simulink model "test_final_sift"  (R2015a)
settings: Solver=ode45  StartTime=0.0  StopTime=10.0  RelTol=1e-3
InitFcn:
  | %% DSPBuilder Start
  | alt_dspbuilder_update_model(bdroot)
  | %% DSPBuilder End
libraries: allblocks_alteradspbuilder2 x2309
(part 14 of 27)

== system test_final_sift/sift_octave1/matching/Ram/picture_first ==
  descriptor : Inport
  eof : Inport  Port=2
  clken : Inport  Port=3
  allow : Inport  Port=4
  AltBus : allblocks_alteradspbuilder2/AltBus  BusType=Unsigned Integer  bwl=1  bwr=0  saturate=off  floatingPointInput=on  floatingPointOutput=on  logOutputs=off  logFile=C:\Users\ASUS\Desktop\sift_fpga\Octave_2\tb_test_final_sift\test%5Ffinal%5Fsift_sift%5Foctave1_matching_Ram_picture%5Ffirst_AltBus.fixedpointlog
  AltBus1 : allblocks_alteradspbuilder2/AltBus  BusType=Unsigned Integer  bwl=1172  bwr=0  saturate=off  floatingPointInput=on  floatingPointOutput=on  logOutputs=off  logFile=C:\Users\ASUS\Desktop\sift_fpga\Octave_2\tb_test_final_sift\test%5Ffinal%5Fsift_sift%5Foctave1_matching_Ram_picture%5Ffirst_AltBus1.fixedpointlog
  Comparator : allblocks_alteradspbuilder2/Comparator  direction=a == b  pipeline_display=0  allowFloatingPointOverride=on  logOutputs=off  logFile=C:\Users\ASUS\Desktop\sift_fpga\Octave_2\tb_test_final_sift\test%5Ffinal%5Fsift_sift%5Foctave1_matching_Ram_picture%5Ffirst_Comparator.fixedpointlog
  Constant1 : allblocks_alteradspbuilder2/Constant  mask_cst=1  BusType=Single Bit  bwl=10  bwr=0  roundMode=Truncate  satMode=Wrap  SpecifyClock=off  allowFloatingPointOverride=on  logOutputs=off  logFile=C:\Users\ASUS\Desktop\sift_fpga\Octave_2\tb_test_final_sift\test%5Ffinal%5Fsift_sift%5Foctave1_matching_Ram_picture%5Ffirst_Constant1.fixedpointlog
  Constant2 : allblocks_alteradspbuilder2/Constant  mask_cst=1  BusType=Unsigned Integer  bwl=10  bwr=0  roundMode=Truncate  satMode=Wrap  SpecifyClock=off  allowFloatingPointOverride=on  logOutputs=off  logFile=C:\Users\ASUS\Desktop\sift_fpga\Octave_2\tb_test_final_sift\test%5Ffinal%5Fsift_sift%5Foctave1_matching_Ram_picture%5Ffirst_Constant2.fixedpointlog
  Constant3 : allblocks_alteradspbuilder2/Constant  mask_cst=1  BusType=Single Bit  bwl=1172  bwr=0  roundMode=Truncate  satMode=Wrap  SpecifyClock=off  allowFloatingPointOverride=on  logOutputs=off  logFile=C:\Users\ASUS\Desktop\sift_fpga\Octave_2\tb_test_final_sift\test%5Ffinal%5Fsift_sift%5Foctave1_matching_Ram_picture%5Ffirst_Constant3.fixedpointlog
  Constant4 : allblocks_alteradspbuilder2/Constant  mask_cst=1998  BusType=Unsigned Integer  bwl=1172  bwr=0  roundMode=Truncate  satMode=Wrap  SpecifyClock=off  allowFloatingPointOverride=on  logOutputs=off  logFile=C:\Users\ASUS\Desktop\sift_fpga\Octave_2\tb_test_final_sift\test%5Ffinal%5Fsift_sift%5Foctave1_matching_Ram_picture%5Ffirst_Constant4.fixedpointlog
  Counter : allblocks_alteradspbuilder2/Counter  BusType=Unsigned Integer  bwl=10  bwr=0  use_modulo=on  modulo=1000  SpecifyClock=off  direction=Increment  use_sload=off  use_sset=off  svalue=1  use_clk_ena=off  use_ena=on  use_sclr=on  pipeline_display=1
  Delay : allblocks_alteradspbuilder2/Delay  pipeline=1  pipeline_display=1  ClockPhase=1  use_ena=on  use_sclr=off  allowFloatingPointOverride=on  logOutputs=off  logFile=C:\Users\ASUS\Desktop\sift_fpga\Octave_2\tb_test_final_sift\test%5Ffinal%5Fsift_sift%5Foctave1_matching_Ram_picture%5Ffirst_Delay.fixedpointlog  use_init=off  reset_value=1
  Delay1 : allblocks_alteradspbuilder2/Delay  pipeline=1  pipeline_display=1  ClockPhase=1  use_ena=on  use_sclr=off  allowFloatingPointOverride=on  logOutputs=off  logFile=C:\Users\ASUS\Desktop\sift_fpga\Octave_2\tb_test_final_sift\test%5Ffinal%5Fsift_sift%5Foctave1_matching_Ram_picture%5Ffirst_Delay1.fixedpointlog  use_init=off  reset_value=1
  Delay2 : allblocks_alteradspbuilder2/Delay  pipeline=1  pipeline_display=1  ClockPhase=1  use_ena=on  use_sclr=off  allowFloatingPointOverride=on  logOutputs=off  logFile=C:\Users\ASUS\Desktop\sift_fpga\Octave_2\tb_test_final_sift\test%5Ffinal%5Fsift_sift%5Foctave1_matching_Ram_picture%5Ffirst_Delay2.fixedpointlog  use_init=off  reset_value=1
  Delay3 : allblocks_alteradspbuilder2/Delay  pipeline=1  pipeline_display=1  ClockPhase=1  use_ena=on  use_sclr=off  allowFloatingPointOverride=on  logOutputs=off  logFile=C:\Users\ASUS\Desktop\sift_fpga\Octave_2\tb_test_final_sift\test%5Ffinal%5Fsift_sift%5Foctave1_matching_Ram_picture%5Ffirst_Delay3.fixedpointlog  use_init=off  reset_value=1
  Delay4 : allblocks_alteradspbuilder2/Delay  pipeline=1  pipeline_display=1  ClockPhase=1  use_ena=on  use_sclr=off  allowFloatingPointOverride=on  logOutputs=off  logFile=C:\Users\ASUS\Desktop\sift_fpga\Octave_2\tb_test_final_sift\test%5Ffinal%5Fsift_sift%5Foctave1_matching_Ram_picture%5Ffirst_Delay4.fixedpointlog  use_init=off  reset_value=1
  Logical Bit Operator : allblocks_alteradspbuilder2/Logical Bit Operator  LogicalOperator=OR  user_inputs=2  pipeline_display=0
  Logical Bit Operator1 : allblocks_alteradspbuilder2/Logical Bit Operator  LogicalOperator=AND  user_inputs=2  pipeline_display=0
  Logical Bit Operator2 : allblocks_alteradspbuilder2/Logical Bit Operator  LogicalOperator=NAND  user_inputs=2  pipeline_display=0
  Logical Bit Operator3 : allblocks_alteradspbuilder2/Logical Bit Operator  LogicalOperator=AND  user_inputs=2  pipeline_display=0
  Logical Bus Operator : allblocks_alteradspbuilder2/Logical Bus Operator  BusType=Unsigned Integer  bwl=1173  bwr=0  LogicalOp_text=Shift Right  mask_value_num=-5  shift_amount=1172  force_sign_ext=off  pipeline_display=0
  Multiplexer : allblocks_alteradspbuilder2/Multiplexer  numInputs=2  pipeline=0  oneHot=off  pipeline_display=0  use_ena=off  use_aclr=off  allowFloatingPointOverride=on  logOutputs=off  logFile=C:\Users\ASUS\Desktop\sift_fpga\Octave_2\tb_test_final_sift\test%5Ffinal%5Fsift_sift%5Foctave1_matching_Ram_picture%5Ffirst_Multiplexer.fixedpointlog
  Multiplexer1 : allblocks_alteradspbuilder2/Multiplexer  numInputs=2  pipeline=0  oneHot=off  pipeline_display=0  use_ena=off  use_aclr=off  allowFloatingPointOverride=on  logOutputs=off  logFile=C:\Users\ASUS\Desktop\sift_fpga\Octave_2\tb_test_final_sift\test%5Ffinal%5Fsift_sift%5Foctave1_matching_Ram_picture%5Ffirst_Multiplexer1.fixedpointlog
  Multiplexer2 : allblocks_alteradspbuilder2/Multiplexer  numInputs=2  pipeline=0  oneHot=off  pipeline_display=0  use_ena=off  use_aclr=off  allowFloatingPointOverride=on  logOutputs=off  logFile=C:\Users\ASUS\Desktop\sift_fpga\Octave_2\tb_test_final_sift\test%5Ffinal%5Fsift_sift%5Foctave1_matching_Ram_picture%5Ffirst_Multiplexer2.fixedpointlog
  Parallel Adder Subtractor : allblocks_alteradspbuilder2/Parallel Adder Subtractor  number_of_inputs=2  direction=+  use_pipeline=on  pipeline_display=1  phase_selection=1  use_ena=on  use_aclr=off  allowFloatingPointOverride=on  logOutputs=off  logFile=C:\Users\ASUS\Desktop\sift_fpga\Octave_2\tb_test_final_sift\test%5Ffinal%5Fsift_sift%5Foctave1_matching_Ram_picture%5Ffirst_Parallel+Adder+Subtractor.fixedpointlog
  data : Outport
  add_write : Outport  Port=2
  ena_write : Outport  Port=3
  wires:
  descriptor/1 -> [descriptor]
  [descriptor] -> Logical Bus Operator/1
  Logical Bus Operator/1 -> AltBus/1
  AltBus/1 -> [isKeyPoint]
  [isKeyPoint] -> Logical Bit Operator/1
  eof/1 -> [eof]
  [eof] -> Delay4/1
  Counter/1 -> [add_write]
  [descriptor] -> AltBus1/1
  AltBus1/1 -> [data]
  [eof] -> Comparator/1
  Constant1/1 -> Comparator/2
  [sel] -> Multiplexer/1
  Multiplexer/1 -> Delay1/1
  Comparator/1 -> [sel]
  [data] -> Multiplexer/2
  Constant4/1 -> Multiplexer/3
  clken/1 -> [clken]
  Delay1/1 -> data/1
  [ena] -> Delay1/2
  [sel] -> Delay3/1
  [add_write] -> Delay/1
  Multiplexer1/1 -> add_write/1
  Delay/1 -> Multiplexer1/2
  [ena] -> Delay/2
  [add_write] -> Parallel Adder Subtractor/1
  Constant2/1 -> Parallel Adder Subtractor/2
  [ena] -> Parallel Adder Subtractor/3
  Parallel Adder Subtractor/1 -> Multiplexer1/3
  [sel] -> Multiplexer2/1
  Multiplexer2/1 -> Delay2/1
  [isKeyPoint] -> Multiplexer2/2
  Constant3/1 -> Multiplexer2/3
  [ena] -> Delay2/2
  Delay3/1 -> Multiplexer1/1
  [ena] -> Delay3/2
  Logical Bit Operator/1 -> Counter/1
  Delay4/1 -> Counter/2, Logical Bit Operator/2
  [ena] -> Delay4/2
  allow/1 -> [allow]
  [allow] -> Logical Bit Operator2/2, Logical Bit Operator2/1
  [clken] -> Logical Bit Operator1/2
  Logical Bit Operator2/1 -> Logical Bit Operator1/1
  Logical Bit Operator1/1 -> [ena]
  Delay2/1 -> Logical Bit Operator3/1
  Logical Bit Operator3/1 -> ena_write/1
  [ena] -> Logical Bit Operator3/2

== system test_final_sift/sift_octave1/matching/Ram/picture_second ==
  descriptor : Inport
  eof : Inport  Port=2
  clken : Inport  Port=3
  allow : Inport  Port=4
  AltBus : allblocks_alteradspbuilder2/AltBus  BusType=Unsigned Integer  bwl=1  bwr=0  saturate=off  floatingPointInput=on  floatingPointOutput=on  logOutputs=off  logFile=C:\Users\ASUS\Desktop\sift_fpga\Octave_2\tb_test_final_sift\test%5Ffinal%5Fsift_sift%5Foctave1_matching_Ram_picture%5Fsecond_AltBus.fixedpointlog
  AltBus1 : allblocks_alteradspbuilder2/AltBus  BusType=Unsigned Integer  bwl=1172  bwr=0  saturate=off  floatingPointInput=on  floatingPointOutput=on  logOutputs=off  logFile=C:\Users\ASUS\Desktop\sift_fpga\Octave_2\tb_test_final_sift\test%5Ffinal%5Fsift_sift%5Foctave1_matching_Ram_picture%5Fsecond_AltBus1.fixedpointlog
  Comparator : allblocks_alteradspbuilder2/Comparator  direction=a == b  pipeline_display=0  allowFloatingPointOverride=on  logOutputs=off  logFile=C:\Users\ASUS\Desktop\sift_fpga\Octave_2\tb_test_final_sift\test%5Ffinal%5Fsift_sift%5Foctave1_matching_Ram_picture%5Fsecond_Comparator.fixedpointlog
  Constant1 : allblocks_alteradspbuilder2/Constant  mask_cst=1  BusType=Single Bit  bwl=10  bwr=0  roundMode=Truncate  satMode=Wrap  SpecifyClock=off  allowFloatingPointOverride=on  logOutputs=off  logFile=C:\Users\ASUS\Desktop\sift_fpga\Octave_2\tb_test_final_sift\test%5Ffinal%5Fsift_sift%5Foctave1_matching_Ram_picture%5Fsecond_Constant1.fixedpointlog
  Constant2 : allblocks_alteradspbuilder2/Constant  mask_cst=1  BusType=Unsigned Integer  bwl=10  bwr=0  roundMode=Truncate  satMode=Wrap  SpecifyClock=off  allowFloatingPointOverride=on  logOutputs=off  logFile=C:\Users\ASUS\Desktop\sift_fpga\Octave_2\tb_test_final_sift\test%5Ffinal%5Fsift_sift%5Foctave1_matching_Ram_picture%5Fsecond_Constant2.fixedpointlog
  Constant3 : allblocks_alteradspbuilder2/Constant  mask_cst=1  BusType=Single Bit  bwl=1172  bwr=0  roundMode=Truncate  satMode=Wrap  SpecifyClock=off  allowFloatingPointOverride=on  logOutputs=off  logFile=C:\Users\ASUS\Desktop\sift_fpga\Octave_2\tb_test_final_sift\test%5Ffinal%5Fsift_sift%5Foctave1_matching_Ram_picture%5Fsecond_Constant3.fixedpointlog
  Constant4 : allblocks_alteradspbuilder2/Constant  mask_cst=1998  BusType=Unsigned Integer  bwl=1172  bwr=0  roundMode=Truncate  satMode=Wrap  SpecifyClock=off  allowFloatingPointOverride=on  logOutputs=off  logFile=C:\Users\ASUS\Desktop\sift_fpga\Octave_2\tb_test_final_sift\test%5Ffinal%5Fsift_sift%5Foctave1_matching_Ram_picture%5Fsecond_Constant4.fixedpointlog
  Counter : allblocks_alteradspbuilder2/Counter  BusType=Unsigned Integer  bwl=10  bwr=0  use_modulo=on  modulo=1000  SpecifyClock=off  direction=Increment  use_sload=off  use_sset=off  svalue=1  use_clk_ena=off  use_ena=on  use_sclr=on  pipeline_display=1
  Delay : allblocks_alteradspbuilder2/Delay  pipeline=1  pipeline_display=1  ClockPhase=1  use_ena=on  use_sclr=off  allowFloatingPointOverride=on  logOutputs=off  logFile=C:\Users\ASUS\Desktop\sift_fpga\Octave_2\tb_test_final_sift\test%5Ffinal%5Fsift_sift%5Foctave1_matching_Ram_picture%5Fsecond_Delay.fixedpointlog  use_init=off  reset_value=1
  Delay1 : allblocks_alteradspbuilder2/Delay  pipeline=1  pipeline_display=1  ClockPhase=1  use_ena=on  use_sclr=off  allowFloatingPointOverride=on  logOutputs=off  logFile=C:\Users\ASUS\Desktop\sift_fpga\Octave_2\tb_test_final_sift\test%5Ffinal%5Fsift_sift%5Foctave1_matching_Ram_picture%5Fsecond_Delay1.fixedpointlog  use_init=off  reset_value=1
  Delay2 : allblocks_alteradspbuilder2/Delay  pipeline=1  pipeline_display=1  ClockPhase=1  use_ena=on  use_sclr=off  allowFloatingPointOverride=on  logOutputs=off  logFile=C:\Users\ASUS\Desktop\sift_fpga\Octave_2\tb_test_final_sift\test%5Ffinal%5Fsift_sift%5Foctave1_matching_Ram_picture%5Fsecond_Delay2.fixedpointlog  use_init=off  reset_value=1
  Delay3 : allblocks_alteradspbuilder2/Delay  pipeline=1  pipeline_display=1  ClockPhase=1  use_ena=on  use_sclr=off  allowFloatingPointOverride=on  logOutputs=off  logFile=C:\Users\ASUS\Desktop\sift_fpga\Octave_2\tb_test_final_sift\test%5Ffinal%5Fsift_sift%5Foctave1_matching_Ram_picture%5Fsecond_Delay3.fixedpointlog  use_init=off  reset_value=1
  Delay4 : allblocks_alteradspbuilder2/Delay  pipeline=1  pipeline_display=1  ClockPhase=1  use_ena=on  use_sclr=off  allowFloatingPointOverride=on  logOutputs=off  logFile=C:\Users\ASUS\Desktop\sift_fpga\Octave_2\tb_test_final_sift\test%5Ffinal%5Fsift_sift%5Foctave1_matching_Ram_picture%5Fsecond_Delay4.fixedpointlog  use_init=off  reset_value=1
  Logical Bit Operator : allblocks_alteradspbuilder2/Logical Bit Operator  LogicalOperator=OR  user_inputs=2  pipeline_display=0
  Logical Bit Operator1 : allblocks_alteradspbuilder2/Logical Bit Operator  LogicalOperator=AND  user_inputs=2  pipeline_display=0
  Logical Bit Operator3 : allblocks_alteradspbuilder2/Logical Bit Operator  LogicalOperator=AND  user_inputs=2  pipeline_display=0
  Logical Bus Operator : allblocks_alteradspbuilder2/Logical Bus Operator  BusType=Unsigned Integer  bwl=1173  bwr=0  LogicalOp_text=Shift Right  mask_value_num=-5  shift_amount=1172  force_sign_ext=off  pipeline_display=0
  Multiplexer : allblocks_alteradspbuilder2/Multiplexer  numInputs=2  pipeline=0  oneHot=off  pipeline_display=0  use_ena=off  use_aclr=off  allowFloatingPointOverride=on  logOutputs=off  logFile=C:\Users\ASUS\Desktop\sift_fpga\Octave_2\tb_test_final_sift\test%5Ffinal%5Fsift_sift%5Foctave1_matching_Ram_picture%5Fsecond_Multiplexer.fixedpointlog
  Multiplexer1 : allblocks_alteradspbuilder2/Multiplexer  numInputs=2  pipeline=0  oneHot=off  pipeline_display=0  use_ena=off  use_aclr=off  allowFloatingPointOverride=on  logOutputs=off  logFile=C:\Users\ASUS\Desktop\sift_fpga\Octave_2\tb_test_final_sift\test%5Ffinal%5Fsift_sift%5Foctave1_matching_Ram_picture%5Fsecond_Multiplexer1.fixedpointlog
  Multiplexer2 : allblocks_alteradspbuilder2/Multiplexer  numInputs=2  pipeline=0  oneHot=off  pipeline_display=0  use_ena=off  use_aclr=off  allowFloatingPointOverride=on  logOutputs=off  logFile=C:\Users\ASUS\Desktop\sift_fpga\Octave_2\tb_test_final_sift\test%5Ffinal%5Fsift_sift%5Foctave1_matching_Ram_picture%5Fsecond_Multiplexer2.fixedpointlog
  Parallel Adder Subtractor : allblocks_alteradspbuilder2/Parallel Adder Subtractor  number_of_inputs=2  direction=+  use_pipeline=on  pipeline_display=1  phase_selection=1  use_ena=on  use_aclr=off  allowFloatingPointOverride=on  logOutputs=off  logFile=C:\Users\ASUS\Desktop\sift_fpga\Octave_2\tb_test_final_sift\test%5Ffinal%5Fsift_sift%5Foctave1_matching_Ram_picture%5Fsecond_Parallel+Adder+Subtractor.fixedpointlog
  data : Outport
  add_write : Outport  Port=2
  ena_write : Outport  Port=3
  wires:
  descriptor/1 -> [descriptor]
  [descriptor] -> Logical Bus Operator/1
  Logical Bus Operator/1 -> AltBus/1
  AltBus/1 -> [isKeyPoint]
  [isKeyPoint] -> Logical Bit Operator/1
  eof/1 -> [eof]
  [eof] -> Delay4/1
  Counter/1 -> [add_write]
  [descriptor] -> AltBus1/1
  AltBus1/1 -> [data]
  [eof] -> Comparator/1
  Constant1/1 -> Comparator/2
  [sel] -> Multiplexer/1
  Multiplexer/1 -> Delay1/1
  Comparator/1 -> [sel]
  [data] -> Multiplexer/2
  Constant4/1 -> Multiplexer/3
  clken/1 -> [clken]
  Delay1/1 -> data/1
  [ena] -> Delay1/2
  [sel] -> Delay3/1
  [add_write] -> Delay/1
  Multiplexer1/1 -> add_write/1
  Delay/1 -> Multiplexer1/2
  [ena] -> Delay/2
  [add_write] -> Parallel Adder Subtractor/1
  Constant2/1 -> Parallel Adder Subtractor/2
  [ena] -> Parallel Adder Subtractor/3
  Parallel Adder Subtractor/1 -> Multiplexer1/3
  [sel] -> Multiplexer2/1
  Multiplexer2/1 -> Delay2/1
  [isKeyPoint] -> Multiplexer2/2
  Constant3/1 -> Multiplexer2/3
  [ena] -> Delay2/2
  Delay3/1 -> Multiplexer1/1
  [ena] -> Delay3/2
  Logical Bit Operator/1 -> Counter/1
  Delay4/1 -> Counter/2, Logical Bit Operator/2
  [ena] -> Delay4/2
  allow/1 -> [allow]
  [allow] -> Logical Bit Operator1/1
  [clken] -> Logical Bit Operator1/2
  Logical Bit Operator1/1 -> [ena]
  Delay2/1 -> Logical Bit Operator3/1
  Logical Bit Operator3/1 -> ena_write/1
  [ena] -> Logical Bit Operator3/2

== system test_final_sift/sift_octave1/matching/compare_descriptor/BusSplitter ==
  descriptor_in : Inport
  AltBus : allblocks_alteradspbuilder2/AltBus  BusType=Unsigned Integer  bwl=1024  bwr=0  saturate=off  floatingPointInput=on  floatingPointOutput=on  logOutputs=off  logFile=C:\Users\ASUS\Desktop\sift_fpga\Octave_2\tb_test_final_sift\test%5Ffinal%5Fsift_sift%5Foctave1_matching_compare%5Fdescriptor_BusSplitter_AltBus.fixedpointlog
  AltBus1 : allblocks_alteradspbuilder2/AltBus  BusType=Unsigned Integer  bwl=896  bwr=0  saturate=off  floatingPointInput=on  floatingPointOutput=on  logOutputs=off  logFile=C:\Users\ASUS\Desktop\sift_fpga\Octave_2\tb_test_final_sift\test%5Ffinal%5Fsift_sift%5Foctave1_matching_compare%5Fdescriptor_BusSplitter_AltBus1.fixedpointlog
  AltBus10 : allblocks_alteradspbuilder2/AltBus  BusType=Unsigned Integer  bwl=128  bwr=0  saturate=off  floatingPointInput=on  floatingPointOutput=on  logOutputs=off  logFile=C:\Users\ASUS\Desktop\sift_fpga\Octave_2\tb_test_final_sift\test%5Ffinal%5Fsift_sift%5Foctave1_matching_compare%5Fdescriptor_BusSplitter_AltBus10.fixedpointlog
  AltBus11 : allblocks_alteradspbuilder2/AltBus  BusType=Unsigned Integer  bwl=128  bwr=0  saturate=off  floatingPointInput=on  floatingPointOutput=on  logOutputs=off  logFile=C:\Users\ASUS\Desktop\sift_fpga\Octave_2\tb_test_final_sift\test%5Ffinal%5Fsift_sift%5Foctave1_matching_compare%5Fdescriptor_BusSplitter_AltBus11.fixedpointlog
  AltBus12 : allblocks_alteradspbuilder2/AltBus  BusType=Unsigned Integer  bwl=128  bwr=0  saturate=off  floatingPointInput=on  floatingPointOutput=on  logOutputs=off  logFile=C:\Users\ASUS\Desktop\sift_fpga\Octave_2\tb_test_final_sift\test%5Ffinal%5Fsift_sift%5Foctave1_matching_compare%5Fdescriptor_BusSplitter_AltBus12.fixedpointlog
  AltBus13 : allblocks_alteradspbuilder2/AltBus  BusType=Unsigned Integer  bwl=128  bwr=0  saturate=off  floatingPointInput=on  floatingPointOutput=on  logOutputs=off  logFile=C:\Users\ASUS\Desktop\sift_fpga\Octave_2\tb_test_final_sift\test%5Ffinal%5Fsift_sift%5Foctave1_matching_compare%5Fdescriptor_BusSplitter_AltBus13.fixedpointlog
  AltBus14 : allblocks_alteradspbuilder2/AltBus  BusType=Unsigned Integer  bwl=16*8*9  bwr=0  saturate=off  floatingPointInput=on  floatingPointOutput=on  logOutputs=off  logFile=C:\Users\ASUS\Desktop\sift_fpga\Octave_2\tb_test_final_sift\test%5Ffinal%5Fsift_sift%5Foctave1_matching_compare%5Fdescriptor_BusSplitter_AltBus14.fixedpointlog
  AltBus15 : allblocks_alteradspbuilder2/AltBus  BusType=Unsigned Integer  bwl=128  bwr=0  saturate=off  floatingPointInput=on  floatingPointOutput=on  logOutputs=off  logFile=C:\Users\ASUS\Desktop\sift_fpga\Octave_2\tb_test_final_sift\test%5Ffinal%5Fsift_sift%5Foctave1_matching_compare%5Fdescriptor_BusSplitter_AltBus15.fixedpointlog
  AltBus16 : allblocks_alteradspbuilder2/AltBus  BusType=Unsigned Integer  bwl=256  bwr=0  saturate=off  floatingPointInput=on  floatingPointOutput=on  logOutputs=off  logFile=C:\Users\ASUS\Desktop\sift_fpga\Octave_2\tb_test_final_sift\test%5Ffinal%5Fsift_sift%5Foctave1_matching_compare%5Fdescriptor_BusSplitter_AltBus16.fixedpointlog
  AltBus2 : allblocks_alteradspbuilder2/AltBus  BusType=Unsigned Integer  bwl=768  bwr=0  saturate=off  floatingPointInput=on  floatingPointOutput=on  logOutputs=off  logFile=C:\Users\ASUS\Desktop\sift_fpga\Octave_2\tb_test_final_sift\test%5Ffinal%5Fsift_sift%5Foctave1_matching_compare%5Fdescriptor_BusSplitter_AltBus2.fixedpointlog
  AltBus3 : allblocks_alteradspbuilder2/AltBus  BusType=Unsigned Integer  bwl=640  bwr=0  saturate=off  floatingPointInput=on  floatingPointOutput=on  logOutputs=off  logFile=C:\Users\ASUS\Desktop\sift_fpga\Octave_2\tb_test_final_sift\test%5Ffinal%5Fsift_sift%5Foctave1_matching_compare%5Fdescriptor_BusSplitter_AltBus3.fixedpointlog
  AltBus4 : allblocks_alteradspbuilder2/AltBus  BusType=Unsigned Integer  bwl=512  bwr=0  saturate=off  floatingPointInput=on  floatingPointOutput=on  logOutputs=off  logFile=C:\Users\ASUS\Desktop\sift_fpga\Octave_2\tb_test_final_sift\test%5Ffinal%5Fsift_sift%5Foctave1_matching_compare%5Fdescriptor_BusSplitter_AltBus4.fixedpointlog
  AltBus5 : allblocks_alteradspbuilder2/AltBus  BusType=Unsigned Integer  bwl=384  bwr=0  saturate=off  floatingPointInput=on  floatingPointOutput=on  logOutputs=off  logFile=C:\Users\ASUS\Desktop\sift_fpga\Octave_2\tb_test_final_sift\test%5Ffinal%5Fsift_sift%5Foctave1_matching_compare%5Fdescriptor_BusSplitter_AltBus5.fixedpointlog
  AltBus6 : allblocks_alteradspbuilder2/AltBus  BusType=Unsigned Integer  bwl=128  bwr=0  saturate=off  floatingPointInput=on  floatingPointOutput=on  logOutputs=off  logFile=C:\Users\ASUS\Desktop\sift_fpga\Octave_2\tb_test_final_sift\test%5Ffinal%5Fsift_sift%5Foctave1_matching_compare%5Fdescriptor_BusSplitter_AltBus6.fixedpointlog
  AltBus7 : allblocks_alteradspbuilder2/AltBus  BusType=Unsigned Integer  bwl=128  bwr=0  saturate=off  floatingPointInput=on  floatingPointOutput=on  logOutputs=off  logFile=C:\Users\ASUS\Desktop\sift_fpga\Octave_2\tb_test_final_sift\test%5Ffinal%5Fsift_sift%5Foctave1_matching_compare%5Fdescriptor_BusSplitter_AltBus7.fixedpointlog
  AltBus8 : allblocks_alteradspbuilder2/AltBus  BusType=Unsigned Integer  bwl=128  bwr=0  saturate=off  floatingPointInput=on  floatingPointOutput=on  logOutputs=off  logFile=C:\Users\ASUS\Desktop\sift_fpga\Octave_2\tb_test_final_sift\test%5Ffinal%5Fsift_sift%5Foctave1_matching_compare%5Fdescriptor_BusSplitter_AltBus8.fixedpointlog
  AltBus9 : allblocks_alteradspbuilder2/AltBus  BusType=Unsigned Integer  bwl=128  bwr=0  saturate=off  floatingPointInput=on  floatingPointOutput=on  logOutputs=off  logFile=C:\Users\ASUS\Desktop\sift_fpga\Octave_2\tb_test_final_sift\test%5Ffinal%5Fsift_sift%5Foctave1_matching_compare%5Fdescriptor_BusSplitter_AltBus9.fixedpointlog
  Logical Bus Operator : allblocks_alteradspbuilder2/Logical Bus Operator  BusType=Unsigned Integer  bwl=1152  bwr=0  LogicalOp_text=Shift Right  mask_value_num=-5  shift_amount=8*128  force_sign_ext=off  pipeline_display=0
  Logical Bus Operator1 : allblocks_alteradspbuilder2/Logical Bus Operator  BusType=Unsigned Integer  bwl=1024  bwr=0  LogicalOp_text=Shift Right  mask_value_num=-5  shift_amount=7*128  force_sign_ext=off  pipeline_display=0
  Logical Bus Operator2 : allblocks_alteradspbuilder2/Logical Bus Operator  BusType=Unsigned Integer  bwl=896  bwr=0  LogicalOp_text=Shift Right  mask_value_num=-5  shift_amount=6*128  force_sign_ext=off  pipeline_display=0
  Logical Bus Operator3 : allblocks_alteradspbuilder2/Logical Bus Operator  BusType=Unsigned Integer  bwl=768  bwr=0  LogicalOp_text=Shift Right  mask_value_num=-5  shift_amount=5*128  force_sign_ext=off  pipeline_display=0
  Logical Bus Operator4 : allblocks_alteradspbuilder2/Logical Bus Operator  BusType=Unsigned Integer  bwl=640  bwr=0  LogicalOp_text=Shift Right  mask_value_num=-5  shift_amount=4*128  force_sign_ext=off  pipeline_display=0
  Logical Bus Operator5 : allblocks_alteradspbuilder2/Logical Bus Operator  BusType=Unsigned Integer  bwl=512  bwr=0  LogicalOp_text=Shift Right  mask_value_num=-5  shift_amount=3*128  force_sign_ext=off  pipeline_display=0
  Logical Bus Operator6 : allblocks_alteradspbuilder2/Logical Bus Operator  BusType=Unsigned Integer  bwl=384  bwr=0  LogicalOp_text=Shift Right  mask_value_num=-5  shift_amount=2*128  force_sign_ext=off  pipeline_display=0
  Logical Bus Operator7 : allblocks_alteradspbuilder2/Logical Bus Operator  BusType=Unsigned Integer  bwl=256  bwr=0  LogicalOp_text=Shift Right  mask_value_num=-5  shift_amount=128  force_sign_ext=off  pipeline_display=0
  hist1 : Outport
  hist2 : Outport  Port=2
  hist3 : Outport  Port=3
  hist4 : Outport  Port=4
  hist5 : Outport  Port=5
  hist6 : Outport  Port=6
  hist7 : Outport  Port=7
  hist8 : Outport  Port=8
  hist9 : Outport  Port=9
  wires:
  Logical Bus Operator6/1 -> AltBus7/1
  AltBus1/1 -> Logical Bus Operator2/1
  AltBus9/1 -> hist5/1
  AltBus8/1 -> hist6/1
  AltBus7/1 -> hist7/1
  AltBus6/1 -> hist8/1
  AltBus/1 -> Logical Bus Operator1/1
  AltBus10/1 -> hist4/1
  AltBus12/1 -> hist3/1
  AltBus11/1 -> hist1/1
  AltBus3/1 -> Logical Bus Operator4/1
  AltBus2/1 -> Logical Bus Operator3/1
  AltBus4/1 -> Logical Bus Operator5/1
  descriptor_in/1 -> AltBus14/1
  AltBus5/1 -> Logical Bus Operator6/1
  Logical Bus Operator1/1 -> AltBus13/1
  Logical Bus Operator2/1 -> AltBus12/1
  Logical Bus Operator/1 -> AltBus11/1
  Logical Bus Operator5/1 -> AltBus8/1
  Logical Bus Operator4/1 -> AltBus9/1
  Logical Bus Operator3/1 -> AltBus10/1
  AltBus13/1 -> hist2/1
  AltBus15/1 -> hist9/1
  AltBus14/1 -> AltBus15/1, AltBus16/1, AltBus5/1, AltBus4/1, AltBus3/1, AltBus2/1, AltBus1/1, AltBus/1, Logical Bus Operator/1
  AltBus16/1 -> Logical Bus Operator7/1
  Logical Bus Operator7/1 -> AltBus6/1

== system test_final_sift/sift_octave1/matching/compare_descriptor/BusSplitter1 ==
  descriptor_in : Inport
  AltBus : allblocks_alteradspbuilder2/AltBus  BusType=Unsigned Integer  bwl=1024  bwr=0  saturate=off  floatingPointInput=on  floatingPointOutput=on  logOutputs=off  logFile=C:\Users\ASUS\Desktop\sift_fpga\Octave_2\tb_test_final_sift\test%5Ffinal%5Fsift_sift%5Foctave1_matching_compare%5Fdescriptor_BusSplitter1_AltBus.fixedpointlog
  AltBus1 : allblocks_alteradspbuilder2/AltBus  BusType=Unsigned Integer  bwl=896  bwr=0  saturate=off  floatingPointInput=on  floatingPointOutput=on  logOutputs=off  logFile=C:\Users\ASUS\Desktop\sift_fpga\Octave_2\tb_test_final_sift\test%5Ffinal%5Fsift_sift%5Foctave1_matching_compare%5Fdescriptor_BusSplitter1_AltBus1.fixedpointlog
  AltBus10 : allblocks_alteradspbuilder2/AltBus  BusType=Unsigned Integer  bwl=128  bwr=0  saturate=off  floatingPointInput=on  floatingPointOutput=on  logOutputs=off  logFile=C:\Users\ASUS\Desktop\sift_fpga\Octave_2\tb_test_final_sift\test%5Ffinal%5Fsift_sift%5Foctave1_matching_compare%5Fdescriptor_BusSplitter1_AltBus10.fixedpointlog
  AltBus11 : allblocks_alteradspbuilder2/AltBus  BusType=Unsigned Integer  bwl=128  bwr=0  saturate=off  floatingPointInput=on  floatingPointOutput=on  logOutputs=off  logFile=C:\Users\ASUS\Desktop\sift_fpga\Octave_2\tb_test_final_sift\test%5Ffinal%5Fsift_sift%5Foctave1_matching_compare%5Fdescriptor_BusSplitter1_AltBus11.fixedpointlog
  AltBus12 : allblocks_alteradspbuilder2/AltBus  BusType=Unsigned Integer  bwl=128  bwr=0  saturate=off  floatingPointInput=on  floatingPointOutput=on  logOutputs=off  logFile=C:\Users\ASUS\Desktop\sift_fpga\Octave_2\tb_test_final_sift\test%5Ffinal%5Fsift_sift%5Foctave1_matching_compare%5Fdescriptor_BusSplitter1_AltBus12.fixedpointlog
  AltBus13 : allblocks_alteradspbuilder2/AltBus  BusType=Unsigned Integer  bwl=128  bwr=0  saturate=off  floatingPointInput=on  floatingPointOutput=on  logOutputs=off  logFile=C:\Users\ASUS\Desktop\sift_fpga\Octave_2\tb_test_final_sift\test%5Ffinal%5Fsift_sift%5Foctave1_matching_compare%5Fdescriptor_BusSplitter1_AltBus13.fixedpointlog
  AltBus14 : allblocks_alteradspbuilder2/AltBus  BusType=Unsigned Integer  bwl=16*8*9  bwr=0  saturate=off  floatingPointInput=on  floatingPointOutput=on  logOutputs=off  logFile=C:\Users\ASUS\Desktop\sift_fpga\Octave_2\tb_test_final_sift\test%5Ffinal%5Fsift_sift%5Foctave1_matching_compare%5Fdescriptor_BusSplitter1_AltBus14.fixedpointlog
  AltBus15 : allblocks_alteradspbuilder2/AltBus  BusType=Unsigned Integer  bwl=128  bwr=0  saturate=off  floatingPointInput=on  floatingPointOutput=on  logOutputs=off  logFile=C:\Users\ASUS\Desktop\sift_fpga\Octave_2\tb_test_final_sift\test%5Ffinal%5Fsift_sift%5Foctave1_matching_compare%5Fdescriptor_BusSplitter1_AltBus15.fixedpointlog
  AltBus16 : allblocks_alteradspbuilder2/AltBus  BusType=Unsigned Integer  bwl=256  bwr=0  saturate=off  floatingPointInput=on  floatingPointOutput=on  logOutputs=off  logFile=C:\Users\ASUS\Desktop\sift_fpga\Octave_2\tb_test_final_sift\test%5Ffinal%5Fsift_sift%5Foctave1_matching_compare%5Fdescriptor_BusSplitter1_AltBus16.fixedpointlog
  AltBus2 : allblocks_alteradspbuilder2/AltBus  BusType=Unsigned Integer  bwl=768  bwr=0  saturate=off  floatingPointInput=on  floatingPointOutput=on  logOutputs=off  logFile=C:\Users\ASUS\Desktop\sift_fpga\Octave_2\tb_test_final_sift\test%5Ffinal%5Fsift_sift%5Foctave1_matching_compare%5Fdescriptor_BusSplitter1_AltBus2.fixedpointlog
  AltBus3 : allblocks_alteradspbuilder2/AltBus  BusType=Unsigned Integer  bwl=640  bwr=0  saturate=off  floatingPointInput=on  floatingPointOutput=on  logOutputs=off  logFile=C:\Users\ASUS\Desktop\sift_fpga\Octave_2\tb_test_final_sift\test%5Ffinal%5Fsift_sift%5Foctave1_matching_compare%5Fdescriptor_BusSplitter1_AltBus3.fixedpointlog
  AltBus4 : allblocks_alteradspbuilder2/AltBus  BusType=Unsigned Integer  bwl=512  bwr=0  saturate=off  floatingPointInput=on  floatingPointOutput=on  logOutputs=off  logFile=C:\Users\ASUS\Desktop\sift_fpga\Octave_2\tb_test_final_sift\test%5Ffinal%5Fsift_sift%5Foctave1_matching_compare%5Fdescriptor_BusSplitter1_AltBus4.fixedpointlog
  AltBus5 : allblocks_alteradspbuilder2/AltBus  BusType=Unsigned Integer  bwl=384  bwr=0  saturate=off  floatingPointInput=on  floatingPointOutput=on  logOutputs=off  logFile=C:\Users\ASUS\Desktop\sift_fpga\Octave_2\tb_test_final_sift\test%5Ffinal%5Fsift_sift%5Foctave1_matching_compare%5Fdescriptor_BusSplitter1_AltBus5.fixedpointlog
  AltBus6 : allblocks_alteradspbuilder2/AltBus  BusType=Unsigned Integer  bwl=128  bwr=0  saturate=off  floatingPointInput=on  floatingPointOutput=on  logOutputs=off  logFile=C:\Users\ASUS\Desktop\sift_fpga\Octave_2\tb_test_final_sift\test%5Ffinal%5Fsift_sift%5Foctave1_matching_compare%5Fdescriptor_BusSplitter1_AltBus6.fixedpointlog
  AltBus7 : allblocks_alteradspbuilder2/AltBus  BusType=Unsigned Integer  bwl=128  bwr=0  saturate=off  floatingPointInput=on  floatingPointOutput=on  logOutputs=off  logFile=C:\Users\ASUS\Desktop\sift_fpga\Octave_2\tb_test_final_sift\test%5Ffinal%5Fsift_sift%5Foctave1_matching_compare%5Fdescriptor_BusSplitter1_AltBus7.fixedpointlog
  AltBus8 : allblocks_alteradspbuilder2/AltBus  BusType=Unsigned Integer  bwl=128  bwr=0  saturate=off  floatingPointInput=on  floatingPointOutput=on  logOutputs=off  logFile=C:\Users\ASUS\Desktop\sift_fpga\Octave_2\tb_test_final_sift\test%5Ffinal%5Fsift_sift%5Foctave1_matching_compare%5Fdescriptor_BusSplitter1_AltBus8.fixedpointlog
  AltBus9 : allblocks_alteradspbuilder2/AltBus  BusType=Unsigned Integer  bwl=128  bwr=0  saturate=off  floatingPointInput=on  floatingPointOutput=on  logOutputs=off  logFile=C:\Users\ASUS\Desktop\sift_fpga\Octave_2\tb_test_final_sift\test%5Ffinal%5Fsift_sift%5Foctave1_matching_compare%5Fdescriptor_BusSplitter1_AltBus9.fixedpointlog
  Logical Bus Operator : allblocks_alteradspbuilder2/Logical Bus Operator  BusType=Unsigned Integer  bwl=1152  bwr=0  LogicalOp_text=Shift Right  mask_value_num=-5  shift_amount=8*128  force_sign_ext=off  pipeline_display=0
  Logical Bus Operator1 : allblocks_alteradspbuilder2/Logical Bus Operator  BusType=Unsigned Integer  bwl=1024  bwr=0  LogicalOp_text=Shift Right  mask_value_num=-5  shift_amount=7*128  force_sign_ext=off  pipeline_display=0
  Logical Bus Operator2 : allblocks_alteradspbuilder2/Logical Bus Operator  BusType=Unsigned Integer  bwl=896  bwr=0  LogicalOp_text=Shift Right  mask_value_num=-5  shift_amount=6*128  force_sign_ext=off  pipeline_display=0
  Logical Bus Operator3 : allblocks_alteradspbuilder2/Logical Bus Operator  BusType=Unsigned Integer  bwl=768  bwr=0  LogicalOp_text=Shift Right  mask_value_num=-5  shift_amount=5*128  force_sign_ext=off  pipeline_display=0
  Logical Bus Operator4 : allblocks_alteradspbuilder2/Logical Bus Operator  BusType=Unsigned Integer  bwl=640  bwr=0  LogicalOp_text=Shift Right  mask_value_num=-5  shift_amount=4*128  force_sign_ext=off  pipeline_display=0
  Logical Bus Operator5 : allblocks_alteradspbuilder2/Logical Bus Operator  BusType=Unsigned Integer  bwl=512  bwr=0  LogicalOp_text=Shift Right  mask_value_num=-5  shift_amount=3*128  force_sign_ext=off  pipeline_display=0
  Logical Bus Operator6 : allblocks_alteradspbuilder2/Logical Bus Operator  BusType=Unsigned Integer  bwl=384  bwr=0  LogicalOp_text=Shift Right  mask_value_num=-5  shift_amount=2*128  force_sign_ext=off  pipeline_display=0
  Logical Bus Operator7 : allblocks_alteradspbuilder2/Logical Bus Operator  BusType=Unsigned Integer  bwl=256  bwr=0  LogicalOp_text=Shift Right  mask_value_num=-5  shift_amount=128  force_sign_ext=off  pipeline_display=0
  hist1 : Outport
  hist2 : Outport  Port=2
  hist3 : Outport  Port=3
  hist4 : Outport  Port=4
  hist5 : Outport  Port=5
  hist6 : Outport  Port=6
  hist7 : Outport  Port=7
  hist8 : Outport  Port=8
  hist9 : Outport  Port=9
  wires:
  Logical Bus Operator6/1 -> AltBus7/1
  AltBus1/1 -> Logical Bus Operator2/1
  AltBus9/1 -> hist5/1
  AltBus8/1 -> hist6/1
  AltBus7/1 -> hist7/1
  AltBus6/1 -> hist8/1
  AltBus/1 -> Logical Bus Operator1/1
  AltBus10/1 -> hist4/1
  AltBus12/1 -> hist3/1
  AltBus11/1 -> hist1/1
  AltBus3/1 -> Logical Bus Operator4/1
  AltBus2/1 -> Logical Bus Operator3/1
  AltBus4/1 -> Logical Bus Operator5/1
  descriptor_in/1 -> AltBus14/1
  AltBus5/1 -> Logical Bus Operator6/1
  Logical Bus Operator1/1 -> AltBus13/1
  Logical Bus Operator2/1 -> AltBus12/1
  Logical Bus Operator/1 -> AltBus11/1
  Logical Bus Operator5/1 -> AltBus8/1
  Logical Bus Operator4/1 -> AltBus9/1
  Logical Bus Operator3/1 -> AltBus10/1
  AltBus13/1 -> hist2/1
  AltBus15/1 -> hist9/1
  AltBus14/1 -> AltBus15/1, AltBus16/1, AltBus5/1, AltBus4/1, AltBus3/1, AltBus2/1, AltBus1/1, AltBus/1, Logical Bus Operator/1
  AltBus16/1 -> Logical Bus Operator7/1
  Logical Bus Operator7/1 -> AltBus6/1

== system test_final_sift/sift_octave1/matching/compare_descriptor/compare ==
  threshold : Inport
  distance : Inport  Port=2
  Comparator : allblocks_alteradspbuilder2/Comparator  direction=a > b  pipeline_display=0  allowFloatingPointOverride=on  logOutputs=off  logFile=C:\Users\ASUS\Desktop\sift_fpga\Octave_2\tb_test_final_sift\test%5Ffinal%5Fsift_sift%5Foctave1_matching_compare%5Fdescriptor_compare_Comparator.fixedpointlog
  match : Outport
  wires:
  threshold/1 -> [threshold]
  distance/1 -> [distance]
  [match] -> match/1
  [threshold] -> Comparator/1
  [distance] -> Comparator/2
  Comparator/1 -> [match]

== system test_final_sift/sift_octave1/matching/compare_descriptor/get_distance ==
  hist_in1 : Inport
  hist_in2 : Inport  Port=2
  clken : Inport  Port=3
  BusSplitter : Subsystem
  BusSplitter1 : Subsystem
  Parallel Adder Subtractor : allblocks_alteradspbuilder2/Parallel Adder Subtractor  number_of_inputs=8  direction=+  use_pipeline=on  pipeline_display=3  phase_selection=1  use_ena=on  use_aclr=off  allowFloatingPointOverride=on  logOutputs=off  logFile=C:\Users\ASUS\Desktop\sift_fpga\Octave_2\tb_test_final_sift\test%5Ffinal%5Fsift_sift%5Foctave1_matching_compare%5Fdescriptor_get%5Fdistance_Parallel+Adder+Subtractor.fixedpointlog
  sub_GradOrian : Subsystem
  sub_GradOrian1 : Subsystem
  sub_GradOrian2 : Subsystem
  sub_GradOrian3 : Subsystem
  sub_GradOrian4 : Subsystem
  sub_GradOrian5 : Subsystem
  sub_GradOrian6 : Subsystem
  sub_GradOrian7 : Subsystem
  distance_out : Outport
  wires:
  hist_in2/1 -> [hist_in2]
  hist_in1/1 -> [hist_in1]
  [hist_in1] -> BusSplitter/1(data_in)
  [hist_in2] -> BusSplitter1/1(data_in)
  BusSplitter/1(bin1) -> [bin_11]
  BusSplitter/2(bin2) -> [bin_12]
  BusSplitter/3(bin3) -> [bin_13]
  BusSplitter/4(bin4) -> [bin_14]
  BusSplitter/5(bin5) -> [bin_15]
  BusSplitter/6(bin6) -> [bin_16]
  BusSplitter/7(bin7) -> [bin_17]
  BusSplitter/8(bin8) -> [bin_18]
  BusSplitter1/1(bin1) -> [bin_21]
  BusSplitter1/2(bin2) -> [bin_22]
  BusSplitter1/3(bin3) -> [bin_23]
  BusSplitter1/4(bin4) -> [bin_24]
  BusSplitter1/5(bin5) -> [bin_25]
  BusSplitter1/6(bin6) -> [bin_26]
  BusSplitter1/7(bin7) -> [bin_27]
  BusSplitter1/8(bin8) -> [bin_28]
  [bin_21] -> sub_GradOrian/2(bin2)
  [bin_11] -> sub_GradOrian/1(bin1)
  clken/1 -> [clken]
  [clken] -> sub_GradOrian/3(clken)
  sub_GradOrian/1(sub_bin) -> [sub_bin1]
  [bin_22] -> sub_GradOrian1/2(bin2)
  [bin_12] -> sub_GradOrian1/1(bin1)
  [clken] -> sub_GradOrian1/3(clken)
  sub_GradOrian1/1(sub_bin) -> [sub_bin2]
  [bin_23] -> sub_GradOrian2/2(bin2)
  [bin_13] -> sub_GradOrian2/1(bin1)
  [clken] -> sub_GradOrian2/3(clken)
  sub_GradOrian2/1(sub_bin) -> [sub_bin3]
  [bin_24] -> sub_GradOrian3/2(bin2)
  [bin_14] -> sub_GradOrian3/1(bin1)
  [clken] -> sub_GradOrian3/3(clken)
  sub_GradOrian3/1(sub_bin) -> [sub_bin4]
  [bin_25] -> sub_GradOrian4/2(bin2)
  [bin_15] -> sub_GradOrian4/1(bin1)
  [clken] -> sub_GradOrian4/3(clken)
  sub_GradOrian4/1(sub_bin) -> [sub_bin5]
  [bin_26] -> sub_GradOrian5/2(bin2)
  [bin_16] -> sub_GradOrian5/1(bin1)
  [clken] -> sub_GradOrian5/3(clken)
  sub_GradOrian5/1(sub_bin) -> [sub_bin6]
  [bin_27] -> sub_GradOrian6/2(bin2)
  [bin_17] -> sub_GradOrian6/1(bin1)
  [clken] -> sub_GradOrian6/3(clken)
  sub_GradOrian6/1(sub_bin) -> [sub_bin7]
  [bin_28] -> sub_GradOrian7/2(bin2)
  [bin_18] -> sub_GradOrian7/1(bin1)
  [clken] -> sub_GradOrian7/3(clken)
  sub_GradOrian7/1(sub_bin) -> [sub_bin8]
  [sub_bin1] -> Parallel Adder Subtractor/1
  [sub_bin2] -> Parallel Adder Subtractor/2
  [sub_bin3] -> Parallel Adder Subtractor/3
  [sub_bin4] -> Parallel Adder Subtractor/4
  [sub_bin5] -> Parallel Adder Subtractor/5
  [sub_bin6] -> Parallel Adder Subtractor/6
  [sub_bin7] -> Parallel Adder Subtractor/7
  [sub_bin8] -> Parallel Adder Subtractor/8
  [clken] -> Parallel Adder Subtractor/9
  Parallel Adder Subtractor/1 -> [distance_out]
  [distance_out] -> distance_out/1

== system test_final_sift/sift_octave1/matching/compare_descriptor/get_distance1 ==
  hist_in1 : Inport
  hist_in2 : Inport  Port=2
  clken : Inport  Port=3
  BusSplitter : Subsystem
  BusSplitter1 : Subsystem
  Parallel Adder Subtractor : allblocks_alteradspbuilder2/Parallel Adder Subtractor  number_of_inputs=8  direction=+  use_pipeline=on  pipeline_display=3  phase_selection=1  use_ena=on  use_aclr=off  allowFloatingPointOverride=on  logOutputs=off  logFile=C:\Users\ASUS\Desktop\sift_fpga\Octave_2\tb_test_final_sift\test%5Ffinal%5Fsift_sift%5Foctave1_matching_compare%5Fdescriptor_get%5Fdistance1_Parallel+Adder+Subtractor.fixedpointlog
  sub_GradOrian : Subsystem
  sub_GradOrian1 : Subsystem
  sub_GradOrian2 : Subsystem
  sub_GradOrian3 : Subsystem
  sub_GradOrian4 : Subsystem
  sub_GradOrian5 : Subsystem
  sub_GradOrian6 : Subsystem
  sub_GradOrian7 : Subsystem
  distance_out : Outport
  wires:
  hist_in2/1 -> [hist_in2]
  hist_in1/1 -> [hist_in1]
  [hist_in1] -> BusSplitter/1(data_in)
  [hist_in2] -> BusSplitter1/1(data_in)
  BusSplitter/1(bin1) -> [bin_11]
  BusSplitter/2(bin2) -> [bin_12]
  BusSplitter/3(bin3) -> [bin_13]
  BusSplitter/4(bin4) -> [bin_14]
  BusSplitter/5(bin5) -> [bin_15]
  BusSplitter/6(bin6) -> [bin_16]
  BusSplitter/7(bin7) -> [bin_17]
  BusSplitter/8(bin8) -> [bin_18]
  BusSplitter1/1(bin1) -> [bin_21]
  BusSplitter1/2(bin2) -> [bin_22]
  BusSplitter1/3(bin3) -> [bin_23]
  BusSplitter1/4(bin4) -> [bin_24]
  BusSplitter1/5(bin5) -> [bin_25]
  BusSplitter1/6(bin6) -> [bin_26]
  BusSplitter1/7(bin7) -> [bin_27]
  BusSplitter1/8(bin8) -> [bin_28]
  [bin_21] -> sub_GradOrian/2(bin2)
  [bin_11] -> sub_GradOrian/1(bin1)
  clken/1 -> [clken]
  [clken] -> sub_GradOrian/3(clken)
  sub_GradOrian/1(sub_bin) -> [sub_bin1]
  [bin_22] -> sub_GradOrian1/2(bin2)
  [bin_12] -> sub_GradOrian1/1(bin1)
  [clken] -> sub_GradOrian1/3(clken)
  sub_GradOrian1/1(sub_bin) -> [sub_bin2]
  [bin_23] -> sub_GradOrian2/2(bin2)
  [bin_13] -> sub_GradOrian2/1(bin1)
  [clken] -> sub_GradOrian2/3(clken)
  sub_GradOrian2/1(sub_bin) -> [sub_bin3]
  [bin_24] -> sub_GradOrian3/2(bin2)
  [bin_14] -> sub_GradOrian3/1(bin1)
  [clken] -> sub_GradOrian3/3(clken)
  sub_GradOrian3/1(sub_bin) -> [sub_bin4]
  [bin_25] -> sub_GradOrian4/2(bin2)
  [bin_15] -> sub_GradOrian4/1(bin1)
  [clken] -> sub_GradOrian4/3(clken)
  sub_GradOrian4/1(sub_bin) -> [sub_bin5]
  [bin_26] -> sub_GradOrian5/2(bin2)
  [bin_16] -> sub_GradOrian5/1(bin1)
  [clken] -> sub_GradOrian5/3(clken)
  sub_GradOrian5/1(sub_bin) -> [sub_bin6]
  [bin_27] -> sub_GradOrian6/2(bin2)
  [bin_17] -> sub_GradOrian6/1(bin1)
  [clken] -> sub_GradOrian6/3(clken)
  sub_GradOrian6/1(sub_bin) -> [sub_bin7]
  [bin_28] -> sub_GradOrian7/2(bin2)
  [bin_18] -> sub_GradOrian7/1(bin1)
  [clken] -> sub_GradOrian7/3(clken)
  sub_GradOrian7/1(sub_bin) -> [sub_bin8]
  [sub_bin1] -> Parallel Adder Subtractor/1
  [sub_bin2] -> Parallel Adder Subtractor/2
  [sub_bin3] -> Parallel Adder Subtractor/3
  [sub_bin4] -> Parallel Adder Subtractor/4
  [sub_bin5] -> Parallel Adder Subtractor/5
  [sub_bin6] -> Parallel Adder Subtractor/6
  [sub_bin7] -> Parallel Adder Subtractor/7
  [sub_bin8] -> Parallel Adder Subtractor/8
  [clken] -> Parallel Adder Subtractor/9
  Parallel Adder Subtractor/1 -> [distance_out]
  [distance_out] -> distance_out/1

== system test_final_sift/sift_octave1/matching/compare_descriptor/get_distance2 ==
  hist_in1 : Inport
  hist_in2 : Inport  Port=2
  clken : Inport  Port=3
  BusSplitter : Subsystem
  BusSplitter1 : Subsystem
  Parallel Adder Subtractor : allblocks_alteradspbuilder2/Parallel Adder Subtractor  number_of_inputs=8  direction=+  use_pipeline=on  pipeline_display=3  phase_selection=1  use_ena=on  use_aclr=off  allowFloatingPointOverride=on  logOutputs=off  logFile=C:\Users\ASUS\Desktop\sift_fpga\Octave_2\tb_test_final_sift\test%5Ffinal%5Fsift_sift%5Foctave1_matching_compare%5Fdescriptor_get%5Fdistance2_Parallel+Adder+Subtractor.fixedpointlog
  sub_GradOrian : Subsystem
  sub_GradOrian1 : Subsystem
  sub_GradOrian2 : Subsystem
  sub_GradOrian3 : Subsystem
  sub_GradOrian4 : Subsystem
  sub_GradOrian5 : Subsystem
  sub_GradOrian6 : Subsystem
  sub_GradOrian7 : Subsystem
  distance_out : Outport
  wires:
  hist_in2/1 -> [hist_in2]
  hist_in1/1 -> [hist_in1]
  [hist_in1] -> BusSplitter/1(data_in)
  [hist_in2] -> BusSplitter1/1(data_in)
  BusSplitter/1(bin1) -> [bin_11]
  BusSplitter/2(bin2) -> [bin_12]
  BusSplitter/3(bin3) -> [bin_13]
  BusSplitter/4(bin4) -> [bin_14]
  BusSplitter/5(bin5) -> [bin_15]
  BusSplitter/6(bin6) -> [bin_16]
  BusSplitter/7(bin7) -> [bin_17]
  BusSplitter/8(bin8) -> [bin_18]
  BusSplitter1/1(bin1) -> [bin_21]
  BusSplitter1/2(bin2) -> [bin_22]
  BusSplitter1/3(bin3) -> [bin_23]
  BusSplitter1/4(bin4) -> [bin_24]
  BusSplitter1/5(bin5) -> [bin_25]
  BusSplitter1/6(bin6) -> [bin_26]
  BusSplitter1/7(bin7) -> [bin_27]
  BusSplitter1/8(bin8) -> [bin_28]
  [bin_21] -> sub_GradOrian/2(bin2)
  [bin_11] -> sub_GradOrian/1(bin1)
  clken/1 -> [clken]
  [clken] -> sub_GradOrian/3(clken)
  sub_GradOrian/1(sub_bin) -> [sub_bin1]
  [bin_22] -> sub_GradOrian1/2(bin2)
  [bin_12] -> sub_GradOrian1/1(bin1)
  [clken] -> sub_GradOrian1/3(clken)
  sub_GradOrian1/1(sub_bin) -> [sub_bin2]
  [bin_23] -> sub_GradOrian2/2(bin2)
  [bin_13] -> sub_GradOrian2/1(bin1)
  [clken] -> sub_GradOrian2/3(clken)
  sub_GradOrian2/1(sub_bin) -> [sub_bin3]
  [bin_24] -> sub_GradOrian3/2(bin2)
  [bin_14] -> sub_GradOrian3/1(bin1)
  [clken] -> sub_GradOrian3/3(clken)
  sub_GradOrian3/1(sub_bin) -> [sub_bin4]
  [bin_25] -> sub_GradOrian4/2(bin2)
  [bin_15] -> sub_GradOrian4/1(bin1)
  [clken] -> sub_GradOrian4/3(clken)
  sub_GradOrian4/1(sub_bin) -> [sub_bin5]
  [bin_26] -> sub_GradOrian5/2(bin2)
  [bin_16] -> sub_GradOrian5/1(bin1)
  [clken] -> sub_GradOrian5/3(clken)
  sub_GradOrian5/1(sub_bin) -> [sub_bin6]
  [bin_27] -> sub_GradOrian6/2(bin2)
  [bin_17] -> sub_GradOrian6/1(bin1)
  [clken] -> sub_GradOrian6/3(clken)
  sub_GradOrian6/1(sub_bin) -> [sub_bin7]
  [bin_28] -> sub_GradOrian7/2(bin2)
  [bin_18] -> sub_GradOrian7/1(bin1)
  [clken] -> sub_GradOrian7/3(clken)
  sub_GradOrian7/1(sub_bin) -> [sub_bin8]
  [sub_bin1] -> Parallel Adder Subtractor/1
  [sub_bin2] -> Parallel Adder Subtractor/2
  [sub_bin3] -> Parallel Adder Subtractor/3
  [sub_bin4] -> Parallel Adder Subtractor/4
  [sub_bin5] -> Parallel Adder Subtractor/5
  [sub_bin6] -> Parallel Adder Subtractor/6
  [sub_bin7] -> Parallel Adder Subtractor/7
  [sub_bin8] -> Parallel Adder Subtractor/8
  [clken] -> Parallel Adder Subtractor/9
  Parallel Adder Subtractor/1 -> [distance_out]
  [distance_out] -> distance_out/1

== system test_final_sift/sift_octave1/matching/compare_descriptor/get_distance3 ==
  hist_in1 : Inport
  hist_in2 : Inport  Port=2
  clken : Inport  Port=3
  BusSplitter : Subsystem
  BusSplitter1 : Subsystem
  Parallel Adder Subtractor : allblocks_alteradspbuilder2/Parallel Adder Subtractor  number_of_inputs=8  direction=+  use_pipeline=on  pipeline_display=3  phase_selection=1  use_ena=on  use_aclr=off  allowFloatingPointOverride=on  logOutputs=off  logFile=C:\Users\ASUS\Desktop\sift_fpga\Octave_2\tb_test_final_sift\test%5Ffinal%5Fsift_sift%5Foctave1_matching_compare%5Fdescriptor_get%5Fdistance3_Parallel+Adder+Subtractor.fixedpointlog
  sub_GradOrian : Subsystem
  sub_GradOrian1 : Subsystem
  sub_GradOrian2 : Subsystem
  sub_GradOrian3 : Subsystem
  sub_GradOrian4 : Subsystem
  sub_GradOrian5 : Subsystem
  sub_GradOrian6 : Subsystem
  sub_GradOrian7 : Subsystem
  distance_out : Outport
  wires:
  hist_in2/1 -> [hist_in2]
  hist_in1/1 -> [hist_in1]
  [hist_in1] -> BusSplitter/1(data_in)
  [hist_in2] -> BusSplitter1/1(data_in)
  BusSplitter/1(bin1) -> [bin_11]
  BusSplitter/2(bin2) -> [bin_12]
  BusSplitter/3(bin3) -> [bin_13]
  BusSplitter/4(bin4) -> [bin_14]
  BusSplitter/5(bin5) -> [bin_15]
  BusSplitter/6(bin6) -> [bin_16]
  BusSplitter/7(bin7) -> [bin_17]
  BusSplitter/8(bin8) -> [bin_18]
  BusSplitter1/1(bin1) -> [bin_21]
  BusSplitter1/2(bin2) -> [bin_22]
  BusSplitter1/3(bin3) -> [bin_23]
  BusSplitter1/4(bin4) -> [bin_24]
  BusSplitter1/5(bin5) -> [bin_25]
  BusSplitter1/6(bin6) -> [bin_26]
  BusSplitter1/7(bin7) -> [bin_27]
  BusSplitter1/8(bin8) -> [bin_28]
  [bin_21] -> sub_GradOrian/2(bin2)
  [bin_11] -> sub_GradOrian/1(bin1)
  clken/1 -> [clken]
  [clken] -> sub_GradOrian/3(clken)
  sub_GradOrian/1(sub_bin) -> [sub_bin1]
  [bin_22] -> sub_GradOrian1/2(bin2)
  [bin_12] -> sub_GradOrian1/1(bin1)
  [clken] -> sub_GradOrian1/3(clken)
  sub_GradOrian1/1(sub_bin) -> [sub_bin2]
  [bin_23] -> sub_GradOrian2/2(bin2)
  [bin_13] -> sub_GradOrian2/1(bin1)
  [clken] -> sub_GradOrian2/3(clken)
  sub_GradOrian2/1(sub_bin) -> [sub_bin3]
  [bin_24] -> sub_GradOrian3/2(bin2)
  [bin_14] -> sub_GradOrian3/1(bin1)
  [clken] -> sub_GradOrian3/3(clken)
  sub_GradOrian3/1(sub_bin) -> [sub_bin4]
  [bin_25] -> sub_GradOrian4/2(bin2)
  [bin_15] -> sub_GradOrian4/1(bin1)
  [clken] -> sub_GradOrian4/3(clken)
  sub_GradOrian4/1(sub_bin) -> [sub_bin5]
  [bin_26] -> sub_GradOrian5/2(bin2)
  [bin_16] -> sub_GradOrian5/1(bin1)
  [clken] -> sub_GradOrian5/3(clken)
  sub_GradOrian5/1(sub_bin) -> [sub_bin6]
  [bin_27] -> sub_GradOrian6/2(bin2)
  [bin_17] -> sub_GradOrian6/1(bin1)
  [clken] -> sub_GradOrian6/3(clken)
  sub_GradOrian6/1(sub_bin) -> [sub_bin7]
  [bin_28] -> sub_GradOrian7/2(bin2)
  [bin_18] -> sub_GradOrian7/1(bin1)
  [clken] -> sub_GradOrian7/3(clken)
  sub_GradOrian7/1(sub_bin) -> [sub_bin8]
  [sub_bin1] -> Parallel Adder Subtractor/1
  [sub_bin2] -> Parallel Adder Subtractor/2
  [sub_bin3] -> Parallel Adder Subtractor/3
  [sub_bin4] -> Parallel Adder Subtractor/4
  [sub_bin5] -> Parallel Adder Subtractor/5
  [sub_bin6] -> Parallel Adder Subtractor/6
  [sub_bin7] -> Parallel Adder Subtractor/7
  [sub_bin8] -> Parallel Adder Subtractor/8
  [clken] -> Parallel Adder Subtractor/9
  Parallel Adder Subtractor/1 -> [distance_out]
  [distance_out] -> distance_out/1
